simulink model "Sim_exercise3_1"  (R2014b)
settings: Solver=VariableStepAuto  StartTime=0.0  StopTime=0.1  RelTol=1e-3
values from neighbouring files (symbols this model uses):
  dm = 3.8E-6    (= 3.8e-06)    [Exercise_2.m]    (also in Exercise_4.m; Exercise_5.m)
  Jeq = Jm + (J1+J2)/(n^2)    (= 2.186e-06)    [Exercise_2.m]    (also in Exercise_4.m; Exercise_5.m = 1.466e-06)
  Kemf = 1/(137*2*pi/60)    (= 0.0697028947848)    [Exercise_2.m]    (also in Exercise_4.m; Exercise_5.m)
  Km = 69.7E-3    (= 0.0697)    [Exercise_2.m]    (also in Exercise_4.m; Exercise_5.m)
  n = 5    [Exercise_2.m]    (also in Exercise_4.m; Exercise_5.m)
  R = 112    [Exercise_2.m]    (also in Exercise_4.m; Exercise_5.m)
  Tc = 1E-3    (= 0.001)    [Exercise_4.m]    (also in Exercise_5.m)
  voltage = 2    [Exercise_4.m]
settings Model: Creator=sofianh  LastModifiedBy=sofianh
settings DataIOCC: SaveFormat=Dataset
settings OptimizationCC: UseDivisionForNetSlopeComputation=off  SimCompilerOptimization=off
settings DebuggingCC: SolverPrmCheckMsg=none  FrameProcessingCompatibilityMsg=error  AllowSymbolicDim=off
settings HardwareCC: ProdBitPerPointer=64  ProdLargestAtomicFloat=Float  ProdIntDivRoundTo=Zero  ProdEndianess=LittleEndian  ProdWordSize=64  ProdHWDeviceType=Intel->x86-64 (Windows64)
settings RTWCC: RTWCompilerOptimization=off
settings GRTTargetCC: GeneratePreprocessorConditionals=Use local settings
settings ConfigComp: CovMetricSettings=dw  CovHtmlReporting=on  CovSaveCumulativeToWorkspaceVar=on  CovSaveSingleToWorkspaceVar=on  CovExternalEMLEnable=off

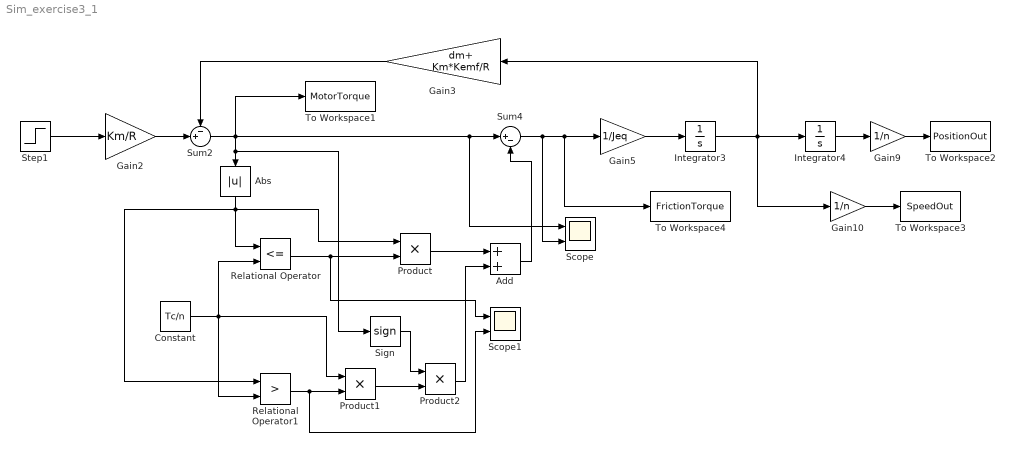
== system Sim_exercise3_1 ==
  Abs : Abs
  Add : Sum
  Constant : Constant  Value=Tc/n
  Gain10 : Gain  Gain=1/n
  Gain2 : Gain  Gain=Km/R
  Gain3 : Gain  Gain=dm+ Km*Kemf/R
  Gain5 : Gain  Gain=1/Jeq
  Gain9 : Gain  Gain=1/n
  Integrator3 : Integrator
  Integrator4 : Integrator
  Product : Product
  Product1 : Product
  Product2 : Product
  Relational Operator : RelationalOperator  Operator=<=  OutDataTypeStr=boolean
  Relational Operator1 : RelationalOperator  Operator=>  OutDataTypeStr=boolean
  Scope : Scope  NumInputPorts=2
      settings: YMin=0.00052~-5  YMax=0.00072~5
  Scope1 : Scope  NumInputPorts=2
      settings: YMin=-8e-05~-5  YMax=0.0007~5
  Sign : Signum
  Step1 : Step  Time=0  After=voltage  SampleTime=0
  Sum2 : Sum  Inputs=-+|
  Sum4 : Sum  Inputs=|+-
  To Workspace1 : ToWorkspace  VariableName=MotorTorque  SaveFormat=Structure With Time  SampleTime=-1
  To Workspace2 : ToWorkspace  VariableName=PositionOut  SaveFormat=Structure With Time  SampleTime=-1
  To Workspace3 : ToWorkspace  VariableName=SpeedOut  SaveFormat=Structure With Time  SampleTime=-1
  To Workspace4 : ToWorkspace  VariableName=FrictionTorque  SaveFormat=Structure With Time  SampleTime=-1
  wires:
  Gain2/1 -> Sum2/2
  Integrator3/1 -> Integrator4/1, Gain10/1, Gain3/1
  Gain3/1 -> Sum2/1
  Relational Operator/1 -> Scope1/1, Product/2
  Sum4/1 -> Scope/2, To Workspace4/1, Gain5/1
  Gain5/1 -> Integrator3/1
  Integrator4/1 -> Gain9/1
  Gain9/1 -> To Workspace2/1
  Gain10/1 -> To Workspace3/1
  Step1/1 -> Gain2/1
  Add/1 -> Sum4/2
  Sum2/1 -> To Workspace1/1, Scope/1, Sum4/1, Sign/1, Abs/1
  Constant/1 -> Relational Operator1/2, Product1/1, Relational Operator/2
  Relational Operator1/1 -> Scope1/2, Product1/2
  Product/1 -> Add/1
  Abs/1 -> Relational Operator1/1, Relational Operator/1, Product/1
  Sign/1 -> Product2/1
  Product1/1 -> Product2/2
  Product2/1 -> Add/2
